simulink library "filckering_filter"  (R2024b)
settings: Solver=VariableStepAuto  StartTime=0.0  StopTime=10.0  RelTol=1e-3
settings Model: Creator=mainuser  LastModifiedBy=mainuser

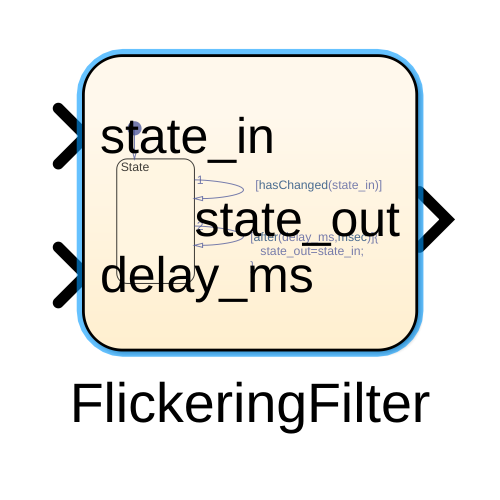
[thumbnail: Simulink's stored preview of the top-level diagram]
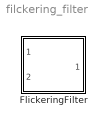
== system filckering_filter ==
  FlickeringFilter : Stateflow chart  TreatAsAtomicUnit=on

== stateflow chart filckering_filter/FlickeringFilter ==
  state State
  (default) -> State
  State -> State [order 1] : [hasChanged(state_in)]
  State -> State [order 2] : [after(delay_ms,msec)]{
      |    state_out=state_in;
      | }
  data: state_in input boolean size=1; state_out output boolean size=1; delay_ms input uint32 size=1
